simulink model "bh_compare_hand_to_SM_quad_pend"  (R2021b)
settings: Solver=ode23t  StartTime=0.0  StopTime=50  FixedStep=0.001  RelTol=1e-5  EnableMultiTasking=on
values from neighbouring files (symbols this model uses):
  K = [0.0865712753524 0.00277244570809 -0.0192153083791 -0.00162453351485 3.32348361895e-08 -1.41900444311e-08 -0.0932413563659 2.38058592401e-06 6.56188614095e-09 -0.0932413743514 2.52459639721e-09 9.53911962763e-08 ... (84 elements, 4x21)]    [CONFIRMED_bh_CONT_DES_RESULTS.mat]    (also in CONFIRMED_bh_CONT_DES_RESULTS_DISCRETE.mat = [-4.44584196463e-19 1.60298866655e-18 6.22915677006e-18 0 -9; CONFIRMED_bh_CONT_DES_RESULTS_DISCRETE_PRE_19a_using_DARE_SOLVER.mat = [-0.000193022438438 0.000285510081841 0.000531074046333 0.00; CONFIRMED_bh_CONT_DES_RESULTS_DISCRETE_R2019b.mat = [3.0073494701e-20 1.31173839205e-18 -5.80308139081e-19 0 8.7; CONFIRMED_bh_CONT_DES_RESULTS_PRE_19a_using_CARE_SOLVER.mat = [3.8473936011e-07 5.10337913269e-05 5.50269068807e-05 0.0072)
  xme_dot_0 = (bRg .') * Vm_0(:)    [bh_func_for_lagr_mask_init.m]
undefined symbols (not defined in the file or in its folder): P_elec, P_mot, P_one_prop, P_pend, P_rot, P_veh, P_veh_no_props, sigbuilder_block, X, Y, Z
libraries: fl_lib x85, simulink_extras x42, nesl_utility x39, sm_lib x29, bh_6dof_LIBRARY x22, slpidlib x8, fl_ps_legacy_lib x7, simulink x2
(part 4 of 5)

== system bh_compare_hand_to_SM_quad_pend/MODEL_SYS/bh_6DOF (Simscape)/6DOF_JOINT_SYS/Angular_MEAS ==
  note: NOTE:  For the Transform sensor  block
      | Tthe DCM is:   r_BASE = R * r_FOLLOWER
  note: NOTE:  For the Transform sensor  block
      | The angular velocities are resolved into FOLLOWER frame components
  Calc Euler_rates : Subsystem
  Gain : Gain
  Math Function : Math  Operator=transpose  SignedPower=on  SaturateOnIntegerOverflow=on
  Mux : Mux  Inputs=3
  PS-Simulink Converter1 : nesl_utility/PS-Simulink Converter  PhysicalDomain=network_engine_domain  SubClassName=ps_output  LeftPortType=input  RightPortType=output  PseudoPeriodic=off  Frequencies=[]  Unit=rad/s  AffineConversion=off
      settings: SourceProductBaseCode=PW,SS
  PS-Simulink Converter2 : nesl_utility/PS-Simulink Converter  PhysicalDomain=network_engine_domain  SubClassName=ps_output  LeftPortType=input  RightPortType=output  PseudoPeriodic=off  Frequencies=[]  Unit=rad/s  AffineConversion=off
      settings: SourceProductBaseCode=PW,SS
  PS-Simulink Converter6 : nesl_utility/PS-Simulink Converter  PhysicalDomain=network_engine_domain  SubClassName=ps_output  LeftPortType=input  RightPortType=output  PseudoPeriodic=off  Frequencies=[]  Unit=1  AffineConversion=off
      settings: SourceProductBaseCode=PW,SS
  PS-Simulink Converter7 : nesl_utility/PS-Simulink Converter  PhysicalDomain=network_engine_domain  SubClassName=ps_output  LeftPortType=input  RightPortType=output  PseudoPeriodic=off  Frequencies=[]  Unit=rad/s  AffineConversion=off
      settings: SourceProductBaseCode=PW,SS
  Reshape1 : Reshape  OutputDimensionality=Column vector (2-D)
  Reshape2 : Reshape  OutputDimensionality=Column vector (2-D)
  Reshape3 : Reshape  OutputDimensionality=Column vector (2-D)
  Transform Sensor : sm_lib/Frames and Transforms/Transform Sensor  MeasurementFrame=Base  SenseAngle=off  SenseAxis=off  SenseAngle1=off  SenseAngle2=off  SenseAngle3=off  SenseQ=off  SenseR=on  SenseOmegaX=off  SenseOmegaY=off  SenseOmegaZ=off  SenseOmega1=off  SenseOmega2=off  SenseOmega3=off  SenseQDot=off  SenseRDot=off  SenseAlphaX=off  SenseAlphaY=off  SenseAlphaZ=off  SenseAlpha1=off  SenseAlpha2=off  SenseAlpha3=off  SenseQDDot=off  SenseRDDot=off  SenseX=off  SenseY=off  SenseZ=off  SenseRad=off  SenseAzim=off  SenseDist=off  SenseInc=off  SenseXDot=off  SenseYDot=off  SenseZDot=off  SenseRadDot=off  SenseAzimDot=off  SenseDistDot=off  SenseIncDot=off  SenseXDDot=off  SenseYDDot=off  SenseZDDot=off  SenseRadDDot=off  SenseAzimDDot=off  SenseDistDDot=off  SenseIncDDot=off
  Transform Sensor1 : sm_lib/Frames and Transforms/Transform Sensor  MeasurementFrame=Follower  SenseAngle=off  SenseAxis=off  SenseAngle1=off  SenseAngle2=off  SenseAngle3=off  SenseQ=off  SenseR=off  SenseOmegaX=on  SenseOmegaY=on  SenseOmegaZ=on  SenseOmega1=off  SenseOmega2=off  SenseOmega3=off  SenseQDot=off  SenseRDot=off  SenseAlphaX=off  SenseAlphaY=off  SenseAlphaZ=off  SenseAlpha1=off  SenseAlpha2=off  SenseAlpha3=off  SenseQDDot=off  SenseRDDot=off  SenseX=off  SenseY=off  SenseZ=off  SenseRad=off  SenseAzim=off  SenseDist=off  SenseInc=off  SenseXDot=off  SenseYDot=off  SenseZDot=off  SenseRadDot=off  SenseAzimDot=off  SenseDistDot=off  SenseIncDot=off  SenseXDDot=off  SenseYDDot=off  SenseZDDot=off  SenseRadDDot=off  SenseAzimDDot=off  SenseDistDDot=off  SenseIncDDot=off
  calc_DCM : MATLAB Function  TreatAsAtomicUnit=on
  B : PMIOPort  Side=Left
  F : PMIOPort  Port=2  Side=Right
  wb : Outport  VectorParamsAs1DForOutWhenUnconnected=off
  bRg : Outport  Port=2  VectorParamsAs1DForOutWhenUnconnected=off
  eul : Outport  Port=3  VectorParamsAs1DForOutWhenUnconnected=off
  eul_rates : Outport  Port=4  VectorParamsAs1DForOutWhenUnconnected=off
  wires:
  PS-Simulink Converter6/1 -> Gain/1  "BRF"
  PS-Simulink Converter7/1 -> Mux/1
  PS-Simulink Converter1/1 -> Mux/2
  PS-Simulink Converter2/1 -> Mux/3
  Gain/1 -> Math Function/1  "gRb"
  Math Function/1 -> [bRg], bRg/1  "bRg"
  Mux/1 -> Reshape1/1
  [bRg] -> calc_DCM/1(bRg)
  calc_DCM/1(eul_vec) -> Reshape2/1
  Reshape2/1 -> [e], eul/1
  Calc Euler_rates/1(Euler_rates) -> Reshape3/1
  Reshape3/1 -> eul_rates/1
  Reshape1/1 -> [wb], wb/1
  [wb] -> Calc Euler_rates/1("p q r ")
  [e] -> Calc Euler_rates/2(Euler_angs)
  connections:
  PS-Simulink Converter7/LConn1 -- Transform Sensor1/RConn2
  PS-Simulink Converter6/LConn1 -- Transform Sensor/RConn2
  Transform Sensor1/RConn1 -- Transform Sensor/RConn1 -- F/RConn1
  Transform Sensor/LConn1 -- B/RConn1 -- Transform Sensor1/LConn1
  PS-Simulink Converter2/LConn1 -- Transform Sensor1/RConn4
  Transform Sensor1/RConn3 -- PS-Simulink Converter1/LConn1

== system bh_compare_hand_to_SM_quad_pend/MODEL_SYS/bh_6DOF (Simscape)/PEND_SYS/Pend_Angular_MEAS ==
  note: NOTE:  For the Transform sensor  block
      | Tthe DCM is:   r_BASE = R * r_FOLLOWER
  note: NOTE:  For the Transform sensor  block
      | The angular velocities are resolved into FOLLOWER frame components
  Calc Euler_rates : Subsystem
  Gain : Gain
  Math Function : Math  Operator=transpose  SignedPower=on  SaturateOnIntegerOverflow=on
  Mux : Mux  Inputs=3
  PS-Simulink Converter1 : nesl_utility/PS-Simulink Converter  PhysicalDomain=network_engine_domain  SubClassName=ps_output  LeftPortType=input  RightPortType=output  PseudoPeriodic=off  Frequencies=[]  Unit=rad/s  AffineConversion=off
      settings: SourceProductBaseCode=PW,SS
  PS-Simulink Converter2 : nesl_utility/PS-Simulink Converter  PhysicalDomain=network_engine_domain  SubClassName=ps_output  LeftPortType=input  RightPortType=output  PseudoPeriodic=off  Frequencies=[]  Unit=rad/s  AffineConversion=off
      settings: SourceProductBaseCode=PW,SS
  PS-Simulink Converter6 : nesl_utility/PS-Simulink Converter  PhysicalDomain=network_engine_domain  SubClassName=ps_output  LeftPortType=input  RightPortType=output  PseudoPeriodic=off  Frequencies=[]  Unit=1  AffineConversion=off
      settings: SourceProductBaseCode=PW,SS
  PS-Simulink Converter7 : nesl_utility/PS-Simulink Converter  PhysicalDomain=network_engine_domain  SubClassName=ps_output  LeftPortType=input  RightPortType=output  PseudoPeriodic=off  Frequencies=[]  Unit=rad/s  AffineConversion=off
      settings: SourceProductBaseCode=PW,SS
  Reshape1 : Reshape  OutputDimensionality=Column vector (2-D)
  Reshape2 : Reshape  OutputDimensionality=Column vector (2-D)
  Reshape3 : Reshape  OutputDimensionality=Column vector (2-D)
  Transform Sensor : sm_lib/Frames and Transforms/Transform Sensor  MeasurementFrame=Base  SenseAngle=off  SenseAxis=off  SenseAngle1=off  SenseAngle2=off  SenseAngle3=off  SenseQ=off  SenseR=on  SenseOmegaX=off  SenseOmegaY=off  SenseOmegaZ=off  SenseOmega1=off  SenseOmega2=off  SenseOmega3=off  SenseQDot=off  SenseRDot=off  SenseAlphaX=off  SenseAlphaY=off  SenseAlphaZ=off  SenseAlpha1=off  SenseAlpha2=off  SenseAlpha3=off  SenseQDDot=off  SenseRDDot=off  SenseX=off  SenseY=off  SenseZ=off  SenseRad=off  SenseAzim=off  SenseDist=off  SenseInc=off  SenseXDot=off  SenseYDot=off  SenseZDot=off  SenseRadDot=off  SenseAzimDot=off  SenseDistDot=off  SenseIncDot=off  SenseXDDot=off  SenseYDDot=off  SenseZDDot=off  SenseRadDDot=off  SenseAzimDDot=off  SenseDistDDot=off  SenseIncDDot=off
  Transform Sensor1 : sm_lib/Frames and Transforms/Transform Sensor  MeasurementFrame=Follower  SenseAngle=off  SenseAxis=off  SenseAngle1=off  SenseAngle2=off  SenseAngle3=off  SenseQ=off  SenseR=off  SenseOmegaX=on  SenseOmegaY=on  SenseOmegaZ=on  SenseOmega1=off  SenseOmega2=off  SenseOmega3=off  SenseQDot=off  SenseRDot=off  SenseAlphaX=off  SenseAlphaY=off  SenseAlphaZ=off  SenseAlpha1=off  SenseAlpha2=off  SenseAlpha3=off  SenseQDDot=off  SenseRDDot=off  SenseX=off  SenseY=off  SenseZ=off  SenseRad=off  SenseAzim=off  SenseDist=off  SenseInc=off  SenseXDot=off  SenseYDot=off  SenseZDot=off  SenseRadDot=off  SenseAzimDot=off  SenseDistDot=off  SenseIncDot=off  SenseXDDot=off  SenseYDDot=off  SenseZDDot=off  SenseRadDDot=off  SenseAzimDDot=off  SenseDistDDot=off  SenseIncDDot=off
      settings: AttributesFormatString=MeasComponentFrame = %<MeasurementFrame>
  calc_DCM : MATLAB Function  TreatAsAtomicUnit=on
  V : PMIOPort  Side=Left
  P : PMIOPort  Port=2  Side=Right
  wb : Outport  VectorParamsAs1DForOutWhenUnconnected=off
  bRg : Outport  Port=2  VectorParamsAs1DForOutWhenUnconnected=off
  eul : Outport  Port=3  VectorParamsAs1DForOutWhenUnconnected=off
  eul_rates : Outport  Port=4  VectorParamsAs1DForOutWhenUnconnected=off
  wires:
  PS-Simulink Converter6/1 -> Gain/1  "BRF"
  PS-Simulink Converter7/1 -> Mux/1
  PS-Simulink Converter1/1 -> Mux/2
  PS-Simulink Converter2/1 -> Mux/3
  Gain/1 -> Math Function/1  "gRb"
  Math Function/1 -> [bRg], bRg/1  "bRg"
  Mux/1 -> Reshape1/1
  [bRg] -> calc_DCM/1(bRg)
  calc_DCM/1(eul_vec) -> Reshape2/1
  Reshape2/1 -> [e], eul/1
  Calc Euler_rates/1(Euler_rates) -> Reshape3/1
  Reshape3/1 -> eul_rates/1
  Reshape1/1 -> [wb], wb/1
  [wb] -> Calc Euler_rates/1("p q r ")
  [e] -> Calc Euler_rates/2(Euler_angs)
  connections:
  PS-Simulink Converter7/LConn1 -- Transform Sensor1/RConn2
  PS-Simulink Converter6/LConn1 -- Transform Sensor/RConn2
  Transform Sensor1/RConn1 -- Transform Sensor/RConn1 -- P/RConn1
  Transform Sensor/LConn1 -- V/RConn1 -- Transform Sensor1/LConn1
  PS-Simulink Converter2/LConn1 -- Transform Sensor1/RConn4
  Transform Sensor1/RConn3 -- PS-Simulink Converter1/LConn1

== system bh_compare_hand_to_SM_quad_pend/MODEL_SYS/bh_6DOF (Simscape)/Propellers/MOT_AERO_PROP_1 ==
  w_CMD_signed : Inport
  Abs : Abs  Commented=on
  Abs1 : Abs  Commented=on
  Bus Creator : BusCreator  Inputs=3
  DRAQ_and_Thrust_on_PROP : Subsystem
  External Force and Torque : sm_lib/Forces and Torques/External Force and Torque  ForceResolutionFrame=AttachedFrame  EnableForceX=off  EnableForceY=off  EnableForceZ=on  EnableForce=off  TorqueResolutionFrame=AttachedFrame  EnableTorqueX=off  EnableTorqueY=off  EnableTorqueZ=on  EnableTorque=off
  From : From  Commented=on  GotoTag=TQ_prop
  From4 : From  Commented=on  GotoTag=TQ_veh
  From5 : From  Commented=on  GotoTag=w_prop
  Gain1 : Gain  Commented=on  Gain=P_mot.b
  Mux : Mux  Commented=on  Inputs=2
  PS-Simulink Converter1 : nesl_utility/PS-Simulink Converter  PhysicalDomain=network_engine_domain  SubClassName=ps_output  LeftPortType=input  RightPortType=output  PseudoPeriodic=off  Frequencies=[]  Unit=rad/s  AffineConversion=off
      settings: SourceProductBaseCode=PW,SS
  PS-Simulink Converter2 : nesl_utility/PS-Simulink Converter  PhysicalDomain=network_engine_domain  SubClassName=ps_output  LeftPortType=input  RightPortType=output  PseudoPeriodic=off  Frequencies=[]  Unit=N*m  AffineConversion=off
      settings: SourceProductBaseCode=PW,SS
  Scope : Scope  Commented=on  NumInputPorts=2
  Selector : Selector  InputPortWidth=3  IndexOptions=Index vector (dialog)  Indices=3  OutputSizes=1
  TQ_on_propeller : Subsystem
  joint_prop : sm_lib/Joints/Revolute Joint  JointMode=Normal  SenseConstraintForce=off  SenseConstraintForceX=off  SenseConstraintForceY=off  SenseConstraintForceZ=off  SenseConstraintTorque=off  SenseConstraintTorqueX=off  SenseConstraintTorqueY=off  SenseConstraintTorqueZ=off  SenseTotalForce=off  SenseTotalForceX=off  SenseTotalForceY=off  SenseTotalForceZ=off  SenseTotalTorque=on  SenseTotalTorqueX=off  SenseTotalTorqueY=off  SenseTotalTorqueZ=off  CompositeWrenchDir=FollowerOnBase  CompositeWrenchFrame=BaseFrame  EquilibriumPosition=0  EquilibriumPositionUnits=deg  SpringStiffness=0  SpringStiffnessUnits=N*m/deg  DampingCoefficient=P_mot.b  DampingCoefficientUnits=N*m/(rad/s)  TorqueActuationMode=InputTorque  MotionActuationMode=ComputedMotion  SensePosition=off  SenseVelocity=on  SenseAcceleration=off  SenseTorqueForce=off  SenseLowerLimitTorqueForce=off  SenseUpperLimitTorqueForce=off  LowerLimitSpecify=off  LowerLimitBound=-90  LowerLimitBoundUnits=deg  LowerLimitStiffness=1e4  LowerLimitStiffnessUnits=N*m/deg  LowerLimitDamping=10  LowerLimitDampingUnits=N*m/(deg/s)  LowerLimitTransitionRegionWidth=0.1  LowerLimitTransitionRegionWidthUnits=deg  UpperLimitSpecify=off  UpperLimitBound=90  UpperLimitBoundUnits=deg  UpperLimitStiffness=1e4  UpperLimitStiffnessUnits=N*m/deg  UpperLimitDamping=10  UpperLimitDampingUnits=N*m/(deg/s)  UpperLimitTransitionRegionWidth=0.1  UpperLimitTransitionRegionWidthUnits=deg  PositionTargetSpecify=off  PositionTargetPriority=High  PositionTargetValue=0  PositionTargetValueUnits=deg  VelocityTargetSpecify=off  VelocityTargetPriority=High  VelocityTargetValue=0  VelocityTargetValueUnits=deg/s
      settings: AttributesFormatString=DAMP = %<DampingCoefficient> %<DampingCoefficientUnits>
  "AirFrame " : PMIOPort  Side=Left
  PROP : PMIOPort  Port=2  Side=Right
  prop_BUS : Outport  VectorParamsAs1DForOutWhenUnconnected=off
  wires:
  w_CMD_signed/1 -> TQ_on_propeller/1(w_CMD_signed)
  TQ_on_propeller/1(TQ_Ki) -> [TQ_prop]
  DRAQ_and_Thrust_on_PROP/1(TH_veh) -> [TH_veh]
  PS-Simulink Converter1/1 -> [w_prop]
  [TH_veh] -> Bus Creator/1  "Thrust_on_veh"
  [w_prop] -> Bus Creator/3  "w_prop"
  [TQ_veh] -> Bus Creator/2  "Torque_on_veh"
  Bus Creator/1 -> prop_BUS/1
  Selector/1 -> [TQ_veh]
  PS-Simulink Converter2/1 -> Selector/1
  Mux/1 -> Scope/1
  From/1 -> Abs1/1
  From4/1 -> Abs/1
  Abs/1 -> Mux/1
  Abs1/1 -> Mux/2
  Gain1/1 -> Scope/2
  From5/1 -> Gain1/1
  connections:
  joint_prop/RConn2 -- DRAQ_and_Thrust_on_PROP/LConn1 -- TQ_on_propeller/LConn1 -- PS-Simulink Converter1/LConn1
  TQ_on_propeller/RConn1 -- joint_prop/LConn2
  External Force and Torque/RConn1 -- joint_prop/RConn1 -- PROP/RConn1
  DRAQ_and_Thrust_on_PROP/RConn2 -- External Force and Torque/LConn2
  DRAQ_and_Thrust_on_PROP/RConn1 -- External Force and Torque/LConn1
  "AirFrame "/RConn1 -- joint_prop/LConn1
  PS-Simulink Converter2/LConn1 -- joint_prop/RConn3

== system bh_compare_hand_to_SM_quad_pend/MODEL_SYS/bh_6DOF (Simscape)/Propellers/MOT_AERO_PROP_2 ==
  w_CMD_signed : Inport
  Abs : Abs  Commented=on
  Abs1 : Abs  Commented=on
  Bus Creator : BusCreator  Inputs=3
  DRAQ_and_Thrust_on_PROP : Subsystem
  External Force and Torque : sm_lib/Forces and Torques/External Force and Torque  ForceResolutionFrame=AttachedFrame  EnableForceX=off  EnableForceY=off  EnableForceZ=on  EnableForce=off  TorqueResolutionFrame=AttachedFrame  EnableTorqueX=off  EnableTorqueY=off  EnableTorqueZ=on  EnableTorque=off
  From : From  Commented=on  GotoTag=TQ_prop
  From4 : From  Commented=on  GotoTag=TQ_veh
  From5 : From  Commented=on  GotoTag=w_prop
  Gain1 : Gain  Commented=on  Gain=P_mot.b
  Mux : Mux  Commented=on  Inputs=2
  PS-Simulink Converter1 : nesl_utility/PS-Simulink Converter  PhysicalDomain=network_engine_domain  SubClassName=ps_output  LeftPortType=input  RightPortType=output  PseudoPeriodic=off  Frequencies=[]  Unit=rad/s  AffineConversion=off
      settings: SourceProductBaseCode=PW,SS
  PS-Simulink Converter2 : nesl_utility/PS-Simulink Converter  PhysicalDomain=network_engine_domain  SubClassName=ps_output  LeftPortType=input  RightPortType=output  PseudoPeriodic=off  Frequencies=[]  Unit=N*m  AffineConversion=off
      settings: SourceProductBaseCode=PW,SS
  Scope : Scope  Commented=on  NumInputPorts=2
  Selector : Selector  InputPortWidth=3  IndexOptions=Index vector (dialog)  Indices=3  OutputSizes=1
  TQ_on_propeller : Subsystem
  joint_prop : sm_lib/Joints/Revolute Joint  JointMode=Normal  SenseConstraintForce=off  SenseConstraintForceX=off  SenseConstraintForceY=off  SenseConstraintForceZ=off  SenseConstraintTorque=off  SenseConstraintTorqueX=off  SenseConstraintTorqueY=off  SenseConstraintTorqueZ=off  SenseTotalForce=off  SenseTotalForceX=off  SenseTotalForceY=off  SenseTotalForceZ=off  SenseTotalTorque=on  SenseTotalTorqueX=off  SenseTotalTorqueY=off  SenseTotalTorqueZ=off  CompositeWrenchDir=FollowerOnBase  CompositeWrenchFrame=BaseFrame  EquilibriumPosition=0  EquilibriumPositionUnits=deg  SpringStiffness=0  SpringStiffnessUnits=N*m/deg  DampingCoefficient=P_mot.b  DampingCoefficientUnits=N*m/(rad/s)  TorqueActuationMode=InputTorque  MotionActuationMode=ComputedMotion  SensePosition=off  SenseVelocity=on  SenseAcceleration=off  SenseTorqueForce=off  SenseLowerLimitTorqueForce=off  SenseUpperLimitTorqueForce=off  LowerLimitSpecify=off  LowerLimitBound=-90  LowerLimitBoundUnits=deg  LowerLimitStiffness=1e4  LowerLimitStiffnessUnits=N*m/deg  LowerLimitDamping=10  LowerLimitDampingUnits=N*m/(deg/s)  LowerLimitTransitionRegionWidth=0.1  LowerLimitTransitionRegionWidthUnits=deg  UpperLimitSpecify=off  UpperLimitBound=90  UpperLimitBoundUnits=deg  UpperLimitStiffness=1e4  UpperLimitStiffnessUnits=N*m/deg  UpperLimitDamping=10  UpperLimitDampingUnits=N*m/(deg/s)  UpperLimitTransitionRegionWidth=0.1  UpperLimitTransitionRegionWidthUnits=deg  PositionTargetSpecify=off  PositionTargetPriority=High  PositionTargetValue=0  PositionTargetValueUnits=deg  VelocityTargetSpecify=off  VelocityTargetPriority=High  VelocityTargetValue=0  VelocityTargetValueUnits=deg/s
      settings: AttributesFormatString=DAMP = %<DampingCoefficient> %<DampingCoefficientUnits>
  "AirFrame " : PMIOPort  Side=Left
  PROP : PMIOPort  Port=2  Side=Right
  prop_BUS : Outport  VectorParamsAs1DForOutWhenUnconnected=off
  wires:
  w_CMD_signed/1 -> TQ_on_propeller/1(w_CMD_signed)
  TQ_on_propeller/1(TQ_Ki) -> [TQ_prop]
  DRAQ_and_Thrust_on_PROP/1(TH_veh) -> [TH_veh]
  PS-Simulink Converter1/1 -> [w_prop]
  [TH_veh] -> Bus Creator/1  "Thrust_on_veh"
  [w_prop] -> Bus Creator/3  "w_prop"
  [TQ_veh] -> Bus Creator/2  "Torque_on_veh"
  Bus Creator/1 -> prop_BUS/1
  Selector/1 -> [TQ_veh]
  PS-Simulink Converter2/1 -> Selector/1
  Mux/1 -> Scope/1
  From/1 -> Abs1/1
  From4/1 -> Abs/1
  Abs/1 -> Mux/1
  Abs1/1 -> Mux/2
  Gain1/1 -> Scope/2
  From5/1 -> Gain1/1
  connections:
  TQ_on_propeller/LConn1 -- PS-Simulink Converter1/LConn1 -- DRAQ_and_Thrust_on_PROP/LConn1 -- joint_prop/RConn2
  TQ_on_propeller/RConn1 -- joint_prop/LConn2
  External Force and Torque/RConn1 -- joint_prop/RConn1 -- PROP/RConn1
  DRAQ_and_Thrust_on_PROP/RConn2 -- External Force and Torque/LConn2
  DRAQ_and_Thrust_on_PROP/RConn1 -- External Force and Torque/LConn1
  "AirFrame "/RConn1 -- joint_prop/LConn1
  PS-Simulink Converter2/LConn1 -- joint_prop/RConn3

== system bh_compare_hand_to_SM_quad_pend/MODEL_SYS/bh_6DOF (Simscape)/Propellers/MOT_AERO_PROP_3 ==
  w_CMD_signed : Inport
  Abs : Abs  Commented=on
  Abs1 : Abs  Commented=on
  Bus Creator : BusCreator  Inputs=3
  DRAQ_and_Thrust_on_PROP : Subsystem
  External Force and Torque : sm_lib/Forces and Torques/External Force and Torque  ForceResolutionFrame=AttachedFrame  EnableForceX=off  EnableForceY=off  EnableForceZ=on  EnableForce=off  TorqueResolutionFrame=AttachedFrame  EnableTorqueX=off  EnableTorqueY=off  EnableTorqueZ=on  EnableTorque=off
  From : From  Commented=on  GotoTag=TQ_prop
  From4 : From  Commented=on  GotoTag=TQ_veh
  From5 : From  Commented=on  GotoTag=w_prop
  Gain1 : Gain  Commented=on  Gain=P_mot.b
  Mux : Mux  Commented=on  Inputs=2
  PS-Simulink Converter1 : nesl_utility/PS-Simulink Converter  PhysicalDomain=network_engine_domain  SubClassName=ps_output  LeftPortType=input  RightPortType=output  PseudoPeriodic=off  Frequencies=[]  Unit=rad/s  AffineConversion=off
      settings: SourceProductBaseCode=PW,SS
  PS-Simulink Converter2 : nesl_utility/PS-Simulink Converter  PhysicalDomain=network_engine_domain  SubClassName=ps_output  LeftPortType=input  RightPortType=output  PseudoPeriodic=off  Frequencies=[]  Unit=N*m  AffineConversion=off
      settings: SourceProductBaseCode=PW,SS
  Scope : Scope  Commented=on  NumInputPorts=2
  Selector : Selector  InputPortWidth=3  IndexOptions=Index vector (dialog)  Indices=3  OutputSizes=1
  TQ_on_propeller : Subsystem
  joint_prop : sm_lib/Joints/Revolute Joint  JointMode=Normal  SenseConstraintForce=off  SenseConstraintForceX=off  SenseConstraintForceY=off  SenseConstraintForceZ=off  SenseConstraintTorque=off  SenseConstraintTorqueX=off  SenseConstraintTorqueY=off  SenseConstraintTorqueZ=off  SenseTotalForce=off  SenseTotalForceX=off  SenseTotalForceY=off  SenseTotalForceZ=off  SenseTotalTorque=on  SenseTotalTorqueX=off  SenseTotalTorqueY=off  SenseTotalTorqueZ=off  CompositeWrenchDir=FollowerOnBase  CompositeWrenchFrame=BaseFrame  EquilibriumPosition=0  EquilibriumPositionUnits=deg  SpringStiffness=0  SpringStiffnessUnits=N*m/deg  DampingCoefficient=P_mot.b  DampingCoefficientUnits=N*m/(rad/s)  TorqueActuationMode=InputTorque  MotionActuationMode=ComputedMotion  SensePosition=off  SenseVelocity=on  SenseAcceleration=off  SenseTorqueForce=off  SenseLowerLimitTorqueForce=off  SenseUpperLimitTorqueForce=off  LowerLimitSpecify=off  LowerLimitBound=-90  LowerLimitBoundUnits=deg  LowerLimitStiffness=1e4  LowerLimitStiffnessUnits=N*m/deg  LowerLimitDamping=10  LowerLimitDampingUnits=N*m/(deg/s)  LowerLimitTransitionRegionWidth=0.1  LowerLimitTransitionRegionWidthUnits=deg  UpperLimitSpecify=off  UpperLimitBound=90  UpperLimitBoundUnits=deg  UpperLimitStiffness=1e4  UpperLimitStiffnessUnits=N*m/deg  UpperLimitDamping=10  UpperLimitDampingUnits=N*m/(deg/s)  UpperLimitTransitionRegionWidth=0.1  UpperLimitTransitionRegionWidthUnits=deg  PositionTargetSpecify=off  PositionTargetPriority=High  PositionTargetValue=0  PositionTargetValueUnits=deg  VelocityTargetSpecify=off  VelocityTargetPriority=High  VelocityTargetValue=0  VelocityTargetValueUnits=deg/s
      settings: AttributesFormatString=DAMP = %<DampingCoefficient> %<DampingCoefficientUnits>
  "AirFrame " : PMIOPort  Side=Left
  PROP : PMIOPort  Port=2  Side=Right
  prop_BUS : Outport  VectorParamsAs1DForOutWhenUnconnected=off
  wires:
  w_CMD_signed/1 -> TQ_on_propeller/1(w_CMD_signed)
  TQ_on_propeller/1(TQ_Ki) -> [TQ_prop]
  DRAQ_and_Thrust_on_PROP/1(TH_veh) -> [TH_veh]
  PS-Simulink Converter1/1 -> [w_prop]
  [TH_veh] -> Bus Creator/1  "Thrust_on_veh"
  [w_prop] -> Bus Creator/3  "w_prop"
  [TQ_veh] -> Bus Creator/2  "Torque_on_veh"
  Bus Creator/1 -> prop_BUS/1
  Selector/1 -> [TQ_veh]
  PS-Simulink Converter2/1 -> Selector/1
  Mux/1 -> Scope/1
  From/1 -> Abs1/1
  From4/1 -> Abs/1
  Abs/1 -> Mux/1
  Abs1/1 -> Mux/2
  Gain1/1 -> Scope/2
  From5/1 -> Gain1/1
  connections:
  TQ_on_propeller/LConn1 -- PS-Simulink Converter1/LConn1 -- DRAQ_and_Thrust_on_PROP/LConn1 -- joint_prop/RConn2
  TQ_on_propeller/RConn1 -- joint_prop/LConn2
  External Force and Torque/RConn1 -- joint_prop/RConn1 -- PROP/RConn1
  DRAQ_and_Thrust_on_PROP/RConn2 -- External Force and Torque/LConn2
  DRAQ_and_Thrust_on_PROP/RConn1 -- External Force and Torque/LConn1
  "AirFrame "/RConn1 -- joint_prop/LConn1
  PS-Simulink Converter2/LConn1 -- joint_prop/RConn3

== system bh_compare_hand_to_SM_quad_pend/MODEL_SYS/bh_6DOF (Simscape)/Propellers/MOT_AERO_PROP_4 ==
  w_CMD_signed : Inport
  Abs : Abs  Commented=on
  Abs1 : Abs  Commented=on
  Bus Creator : BusCreator  Inputs=3
  DRAQ_and_Thrust_on_PROP : Subsystem
  External Force and Torque : sm_lib/Forces and Torques/External Force and Torque  ForceResolutionFrame=AttachedFrame  EnableForceX=off  EnableForceY=off  EnableForceZ=on  EnableForce=off  TorqueResolutionFrame=AttachedFrame  EnableTorqueX=off  EnableTorqueY=off  EnableTorqueZ=on  EnableTorque=off
  From : From  Commented=on  GotoTag=TQ_prop
  From4 : From  Commented=on  GotoTag=TQ_veh
  From5 : From  Commented=on  GotoTag=w_prop
  Gain1 : Gain  Commented=on  Gain=P_mot.b
  Mux : Mux  Commented=on  Inputs=2
  PS-Simulink Converter1 : nesl_utility/PS-Simulink Converter  PhysicalDomain=network_engine_domain  SubClassName=ps_output  LeftPortType=input  RightPortType=output  PseudoPeriodic=off  Frequencies=[]  Unit=rad/s  AffineConversion=off
      settings: SourceProductBaseCode=PW,SS
  PS-Simulink Converter2 : nesl_utility/PS-Simulink Converter  PhysicalDomain=network_engine_domain  SubClassName=ps_output  LeftPortType=input  RightPortType=output  PseudoPeriodic=off  Frequencies=[]  Unit=N*m  AffineConversion=off
      settings: SourceProductBaseCode=PW,SS
  Scope : Scope  Commented=on  NumInputPorts=2
  Selector : Selector  InputPortWidth=3  IndexOptions=Index vector (dialog)  Indices=3  OutputSizes=1
  TQ_on_propeller : Subsystem
  joint_prop : sm_lib/Joints/Revolute Joint  JointMode=Normal  SenseConstraintForce=off  SenseConstraintForceX=off  SenseConstraintForceY=off  SenseConstraintForceZ=off  SenseConstraintTorque=off  SenseConstraintTorqueX=off  SenseConstraintTorqueY=off  SenseConstraintTorqueZ=off  SenseTotalForce=off  SenseTotalForceX=off  SenseTotalForceY=off  SenseTotalForceZ=off  SenseTotalTorque=on  SenseTotalTorqueX=off  SenseTotalTorqueY=off  SenseTotalTorqueZ=off  CompositeWrenchDir=FollowerOnBase  CompositeWrenchFrame=BaseFrame  EquilibriumPosition=0  EquilibriumPositionUnits=deg  SpringStiffness=0  SpringStiffnessUnits=N*m/deg  DampingCoefficient=P_mot.b  DampingCoefficientUnits=N*m/(rad/s)  TorqueActuationMode=InputTorque  MotionActuationMode=ComputedMotion  SensePosition=off  SenseVelocity=on  SenseAcceleration=off  SenseTorqueForce=off  SenseLowerLimitTorqueForce=off  SenseUpperLimitTorqueForce=off  LowerLimitSpecify=off  LowerLimitBound=-90  LowerLimitBoundUnits=deg  LowerLimitStiffness=1e4  LowerLimitStiffnessUnits=N*m/deg  LowerLimitDamping=10  LowerLimitDampingUnits=N*m/(deg/s)  LowerLimitTransitionRegionWidth=0.1  LowerLimitTransitionRegionWidthUnits=deg  UpperLimitSpecify=off  UpperLimitBound=90  UpperLimitBoundUnits=deg  UpperLimitStiffness=1e4  UpperLimitStiffnessUnits=N*m/deg  UpperLimitDamping=10  UpperLimitDampingUnits=N*m/(deg/s)  UpperLimitTransitionRegionWidth=0.1  UpperLimitTransitionRegionWidthUnits=deg  PositionTargetSpecify=off  PositionTargetPriority=High  PositionTargetValue=0  PositionTargetValueUnits=deg  VelocityTargetSpecify=off  VelocityTargetPriority=High  VelocityTargetValue=0  VelocityTargetValueUnits=deg/s
      settings: AttributesFormatString=DAMP = %<DampingCoefficient> %<DampingCoefficientUnits>
  "AirFrame " : PMIOPort  Side=Left
  PROP : PMIOPort  Port=2  Side=Right
  prop_BUS : Outport  VectorParamsAs1DForOutWhenUnconnected=off
  wires:
  w_CMD_signed/1 -> TQ_on_propeller/1(w_CMD_signed)
  TQ_on_propeller/1(TQ_Ki) -> [TQ_prop]
  DRAQ_and_Thrust_on_PROP/1(TH_veh) -> [TH_veh]
  PS-Simulink Converter1/1 -> [w_prop]
  [TH_veh] -> Bus Creator/1  "Thrust_on_veh"
  [w_prop] -> Bus Creator/3  "w_prop"
  [TQ_veh] -> Bus Creator/2  "Torque_on_veh"
  Bus Creator/1 -> prop_BUS/1
  Selector/1 -> [TQ_veh]
  PS-Simulink Converter2/1 -> Selector/1
  Mux/1 -> Scope/1
  From/1 -> Abs1/1
  From4/1 -> Abs/1
  Abs/1 -> Mux/1
  Abs1/1 -> Mux/2
  Gain1/1 -> Scope/2
  From5/1 -> Gain1/1
  connections:
  TQ_on_propeller/LConn1 -- PS-Simulink Converter1/LConn1 -- joint_prop/RConn2 -- DRAQ_and_Thrust_on_PROP/LConn1
  TQ_on_propeller/RConn1 -- joint_prop/LConn2
  External Force and Torque/RConn1 -- joint_prop/RConn1 -- PROP/RConn1
  External Force and Torque/LConn2 -- DRAQ_and_Thrust_on_PROP/RConn2
  External Force and Torque/LConn1 -- DRAQ_and_Thrust_on_PROP/RConn1
  "AirFrame "/RConn1 -- joint_prop/LConn1
  PS-Simulink Converter2/LConn1 -- joint_prop/RConn3

== system bh_compare_hand_to_SM_quad_pend/MODEL_SYS/bh_6DOF (Simscape)/6DOF_JOINT_SYS/Angular_MEAS/Calc Euler_rates ==
  "p q r " : Inport
  Euler_angs : Inport  Port=2
  Demux1 : Demux  Outputs=3
  Demux2 : Demux  Outputs=3
  Demux3 : Demux  Outputs=3
  Mux1 : Mux  Inputs=3
  Reshape1 : Reshape  OutputDimensionality=Column vector (2-D)
  Reshape2 : Reshape  OutputDimensionality=Column vector (2-D)
  Terminator : Terminator
  my_euler_rates : MATLAB Function  TreatAsAtomicUnit=on
  Euler_rates : Outport  VectorParamsAs1DForOutWhenUnconnected=off
  wires:
  Reshape1/1 -> Demux3/1  "wb"
  my_euler_rates/1(euler_rates) -> Demux2/1  "euler_rates"
  Demux2/3 -> Mux1/3  "psidot_X3_roll"
  Demux2/2 -> Mux1/2  "thetadot_Y2_pitch"
  Demux2/1 -> Mux1/1  "phidot_Z1_yaw"
  Reshape2/1 -> Euler_rates/1
  Mux1/1 -> Reshape2/1
  Demux3/3 -> my_euler_rates/5(r)
  Demux3/2 -> my_euler_rates/4(q)
  Demux3/1 -> my_euler_rates/3(p)
  Euler_angs/1 -> Demux1/1
  "p q r "/1 -> Reshape1/1
  Demux1/2 -> my_euler_rates/1(theta)  "theta"
  Demux1/1 -> Terminator/1  "phi"
  Demux1/3 -> my_euler_rates/2(psi)  "psi"

== system bh_compare_hand_to_SM_quad_pend/MODEL_SYS/bh_6DOF (Simscape)/PEND_SYS/Pend_Angular_MEAS/Calc Euler_rates ==
  "p q r " : Inport
  Euler_angs : Inport  Port=2
  Demux1 : Demux  Outputs=3
  Demux2 : Demux  Outputs=3
  Demux3 : Demux  Outputs=3
  Mux1 : Mux  Inputs=3
  Reshape1 : Reshape  OutputDimensionality=Column vector (2-D)
  Reshape2 : Reshape  OutputDimensionality=Column vector (2-D)
  Terminator : Terminator
  my_euler_rates : MATLAB Function  TreatAsAtomicUnit=on
  Euler_rates : Outport  VectorParamsAs1DForOutWhenUnconnected=off
  wires:
  Reshape1/1 -> Demux3/1  "wb"
  my_euler_rates/1(euler_rates) -> Demux2/1  "euler_rates"
  Demux2/3 -> Mux1/3  "psidot_X3_roll"
  Demux2/2 -> Mux1/2  "thetadot_Y2_pitch"
  Demux2/1 -> Mux1/1  "phidot_Z1_yaw"
  Reshape2/1 -> Euler_rates/1
  Mux1/1 -> Reshape2/1
  Demux3/3 -> my_euler_rates/5(r)
  Demux3/2 -> my_euler_rates/4(q)
  Demux3/1 -> my_euler_rates/3(p)
  Euler_angs/1 -> Demux1/1
  "p q r "/1 -> Reshape1/1
  Demux1/2 -> my_euler_rates/1(theta)  "theta"
  Demux1/1 -> Terminator/1  "phi"
  Demux1/3 -> my_euler_rates/2(psi)  "psi"

== system bh_compare_hand_to_SM_quad_pend/MODEL_SYS/bh_6DOF (Simscape)/Propellers/MOT_AERO_PROP_1/DRAQ_and_Thrust_on_PROP ==
  note: The "-1" is because DRAG is in the opposite direction
      | to the propeller SPIN direction
  PS Gain : fl_lib/Physical Signals/Functions/PS Gain  gain=-1
      settings: AttributesFormatString=GAIN= %<gain>
  PS Gain1 : fl_lib/Physical Signals/Functions/PS Gain  gain=P_one_prop.TWIST_per_w2 N*m/((rad/s)^2)
      settings: AttributesFormatString=GAIN= %<gain>
  PS Gain3 : fl_lib/Physical Signals/Functions/PS Gain  gain=P_one_prop.LIFT_per_w2 N/((rad/s)^2)
      settings: AttributesFormatString=GAIN= %<gain>
  PS Product : fl_lib/Physical Signals/Functions/PS Product
  PS Product1 : fl_lib/Physical Signals/Functions/PS Product
  PS Product2 : fl_lib/Physical Signals/Functions/PS Product
  PS Sign : fl_lib/Physical Signals/Nonlinear Operators/PS Sign
      settings: SourceProductBaseCode=SS  InternalSimscapePortConfiguration="{\"Bottom\":[],\"Left\":[{\"id\":\"I\",\"label\":\"\",\"type\":\"input\"}],\"Right\":[{\"id\":\"O\",\"label\":\"\",\"type\":\"output\"}],\"Top\":[]}"
  PS-Simulink Converter1 : nesl_utility/PS-Simulink Converter  PhysicalDomain=network_engine_domain  SubClassName=ps_output  LeftPortType=input  RightPortType=output  PseudoPeriodic=off  Frequencies=[]  Unit=N  AffineConversion=off
      settings: SourceProductBaseCode=PW,SS
  W : PMIOPort  Side=Left
  THRUST : PMIOPort  Port=2  Side=Right
  DRAQ_TQ : PMIOPort  Port=3  Side=Right
  TH_veh : Outport  VectorParamsAs1DForOutWhenUnconnected=off
  wires:
  PS-Simulink Converter1/1 -> TH_veh/1
  connections:
  PS Gain/LConn1 -- PS Sign/RConn1
  W/RConn1 -- PS Product/LConn1 -- PS Product/LConn2 -- PS Product2/LConn1 -- PS Product2/LConn2 -- PS Sign/LConn1
  PS Product/RConn1 -- PS Gain1/LConn1
  PS Gain1/RConn1 -- PS Product1/LConn2
  PS Gain/RConn1 -- PS Product1/LConn1
  DRAQ_TQ/RConn1 -- PS Product1/RConn1
  PS Product2/RConn1 -- PS Gain3/LConn1
  THRUST/RConn1 -- PS Gain3/RConn1 -- PS-Simulink Converter1/LConn1

== system bh_compare_hand_to_SM_quad_pend/MODEL_SYS/bh_6DOF (Simscape)/Propellers/MOT_AERO_PROP_1/TQ_on_propeller ==
  note: ATTENTION:
      | This subsystem computes the Torque that is applied to the
      | PROPELLER ... and NOT the torque applied to the airframe
  w_CMD_signed : Inport
  DC_mot_elec : Subsystem  mask(DC motor){K=P_mot.Ka, R=P_mot.R, L=P_mot.L, Kb=P_mot.Ke, ID=P_mot.ID}
      mask prompts: K "Torque constant (N.m/A)"; R "Armature resistance (ohms)"; L "Armature Inductance (Henry)"; Kb "Back Emf constant (V.sec/rad)"; ID "Motor_ID  (#1 to #4)"
      mask help: DC motor
      mask DialogControl Container4 Prompt: Mechanical
      mask DialogControl Container9 Prompt: Electrical
      mask DialogControl Container32 Prompt: ID
      mask Display: disp('DC motor')
  DC_mot_elec1 : Subsystem  Commented=on  mask(DC motor){K=P_mot.Ka, R=P_mot.R, L=P_mot.L, Kb=P_mot.Ke, ID=P_mot.ID}
      mask prompts: K "Torque constant (N.m/A)"; R "Armature resistance (ohms)"; L "Armature Inductance (Henry)"; Kb "Back Emf constant (V.sec/rad)"; ID "Motor_ID  (#1 to #4)"
      mask help: DC motor
      mask DialogControl Container4 Prompt: Mechanical
      mask DialogControl Container9 Prompt: Electrical
      mask DialogControl Container32 Prompt: ID
      mask Display: disp('DC motor')
  Mux1 : Mux  Inputs=2
  PI_CONT : slpidlib/PID Controller  Controller=PI  Form=Parallel  TimeDomain=Continuous-time  UseExternalTs=off  SampleTime=-1  IntegratorMethod=Forward Euler  FilterMethod=Forward Euler  ControllerParametersSource=internal  P=2.97678216835849  I=24.9655384194189  D=-0.0417302954853434  UseFilter=on  N=6.67624174583517  TunerSelectOption=Transfer Function Based (PID Tuner App)  InitialConditionSource=internal  InitialConditionForIntegrator=0  InitialConditionForFilter=0  DifferentiatorICPrevScaledInput=0  ExternalReset=none  TrackingMode=off  Kt=1  LimitOutput=off  SatLimitsSource=internal  UpperSaturationLimit=inf  LowerSaturationLimit=-inf  LinearizeAsGain=on  AntiWindupMode=none  Kb=1  POutMin=[]  POutMax=[]  IOutMin=[]  IOutMax=[]  DOutMin=[]  DOutMax=[]  NOutMin=[]  NOutMax=[]  SumOutMin=[]  SumOutMax=[]  SaturationOutMin=[]  SaturationOutMax=[]  PParamMin=[]  PParamMax=[]  IParamMin=[]  IParamMax=[]  DParamMin=[]  DParamMax=[]  NParamMin=[]  NParamMax=[]  KbParamMin=[]  KbParamMax=[]  KtParamMin=[]  KtParamMax=[]  KbOutMin=[]  KbOutMax=[]  KtOutMin=[]  KtOutMax=[]  IntegratorOutMin=[]  IntegratorOutMax=[]  FilterOutMin=[]  FilterOutMax=[]  SumI1OutMin=[]  SumI1OutMax=[]  SumI2OutMin=[]  SumI2OutMax=[]  SumI3OutMin=[]  SumI3OutMax=[]  SumI4OutMin=[]  SumI4OutMax=[]  SumDOutMin=[]  SumDOutMax=[]  DifferentiatorOutMin=[]  DifferentiatorOutMax=[]  FilterDiffOutCoefMin=[]  FilterDiffOutCoefMax=[]  ReciprocalOutMin=[]  ReciprocalOutMax=[]  SumDenOutMin=[]  SumDenOutMax=[]  SumNumOutMin=[]  SumNumOutMax=[]  DivideOutMin=[]  DivideOutMax=[]  UdiffTsProdOutMin=[]  UdiffTsProdOutMax=[]  NTsProdOutMin=[]  NTsProdOutMax=[]  UintegralTsProdOutMin=[]  UintegralTsProdOutMax=[]  UngainTsProdOutMin=[]  UngainTsProdOutMax=[]  IntegratorContinuousStateAttributes=''  IntegratorStateMustResolveToSignalObject=off  IntegratorRTWStateStorageClass=Auto  FilterContinuousStateAttributes=''  FilterStateMustResolveToSignalObject=off  FilterRTWStateStorageClass=Auto  ParallelPVariant=InternalParameters  IdealPVariant=Disabled  IVariant=InternalParameters  DVariant=Disabled  IntegratorVariant=Continuous  SatVariant=Disabled  AWVariant=Passthrough  PCopyVariant=Disabled  TRVariant=Disabled  FdbkBlocksVariant=Forward  IdealPFdbkVariant=Disabled  SatFdbkVariant=Disabled  DerivativeFilterVariant=Disabled  NVariant=Disabled  NCopyVariant=Disabled_SignalSpec  FilterICVariant=Disabled  IntegratorICVariant=InternalICs  ExternalResetVariant=Disabled  TRSumVariant=Passthrough  SumFdbkVariant=Disabled  SumVariant=Sum_PI  TsampFilterVariant=InternalTs  TsampNgainVariant=Passthrough  TsampIntegralVariant=Passthrough  ExternalSaturationOutDataTypeStr=Inherit: Same as second input
  PS-Simulink Converter : nesl_utility/PS-Simulink Converter  PhysicalDomain=network_engine_domain  SubClassName=ps_output  LeftPortType=input  RightPortType=output  PseudoPeriodic=off  Frequencies=[]  Unit=rad/s  AffineConversion=off
      settings: SourceProductBaseCode=PW,SS
  PS-Simulink Converter1 : nesl_utility/PS-Simulink Converter  PhysicalDomain=network_engine_domain  SubClassName=ps_output  LeftPortType=input  RightPortType=output  PseudoPeriodic=off  Frequencies=[]  Unit=N*m  AffineConversion=off
      settings: SourceProductBaseCode=PW,SS
  Scope : Scope
  Simulink-PS Converter2 : nesl_utility/Simulink-PS Converter  PhysicalDomain=network_engine_domain  SubClassName=ps_input  LeftPortType=input  RightPortType=output  PseudoPeriodic=off  Frequencies=[]  NoiseDistribution=none  NoiseParameters=[]  Unit=V  AffineConversion=off  FilteringAndDerivatives=provide  SimscapeFilterOrder=1  InputFilterTimeConstant=0.001  UdotUserProvided=0
      settings: SourceProductBaseCode=PW,SS
  Sum1 : Sum  Inputs=|+-
  VOLTAGE Saturation : Saturate  UpperLimit=P_elec.V_mot_max  LowerLimit=P_elec.V_mot_min
      settings: AttributesFormatString=|
      | Vmax = %<UpperLimit>
      | Vmin = %<LowerLimit>
  VOLTS : Scope
  Ki : PMIOPort  Side=Right
  W_MEAS : PMIOPort  Port=2  Side=Left
  TQ_Ki : Outport  VectorParamsAs1DForOutWhenUnconnected=off
  wires:
  VOLTAGE Saturation/1 -> Simulink-PS Converter2/1, VOLTS/1  "VOLTS"
  Sum1/1 -> PI_CONT/1
  PI_CONT/1 -> VOLTAGE Saturation/1  "VOLTS"
  w_CMD_signed/1 -> Sum1/1, [w_signed]  "w_rad_per_sec"
  PS-Simulink Converter/1 -> [wM], Sum1/2
  PS-Simulink Converter1/1 -> TQ_Ki/1
  Mux1/1 -> Scope/1
  [w_signed] -> Mux1/1
  [wM] -> Mux1/2
  connections:
  Simulink-PS Converter2/RConn1 -- DC_mot_elec/LConn1
  PS-Simulink Converter1/LConn1 -- Ki/RConn1 -- DC_mot_elec/RConn1
  W_MEAS/RConn1 -- DC_mot_elec/LConn2 -- PS-Simulink Converter/LConn1

== system bh_compare_hand_to_SM_quad_pend/MODEL_SYS/bh_6DOF (Simscape)/Propellers/MOT_AERO_PROP_2/DRAQ_and_Thrust_on_PROP ==
  note: The "-1" is because DRAG is in the opposite direction
      | to the propeller SPIN direction
  PS Gain : fl_lib/Physical Signals/Functions/PS Gain  gain=-1
      settings: AttributesFormatString=GAIN= %<gain>
  PS Gain1 : fl_lib/Physical Signals/Functions/PS Gain  gain=P_one_prop.TWIST_per_w2 N*m/((rad/s)^2)
      settings: AttributesFormatString=GAIN= %<gain>
  PS Gain3 : fl_lib/Physical Signals/Functions/PS Gain  gain=P_one_prop.LIFT_per_w2 N/((rad/s)^2)
      settings: AttributesFormatString=GAIN= %<gain>
  PS Product : fl_lib/Physical Signals/Functions/PS Product
  PS Product1 : fl_lib/Physical Signals/Functions/PS Product
  PS Product2 : fl_lib/Physical Signals/Functions/PS Product
  PS Sign : fl_lib/Physical Signals/Nonlinear Operators/PS Sign
      settings: SourceProductBaseCode=SS  InternalSimscapePortConfiguration="{\"Bottom\":[],\"Left\":[{\"id\":\"I\",\"label\":\"\",\"type\":\"input\"}],\"Right\":[{\"id\":\"O\",\"label\":\"\",\"type\":\"output\"}],\"Top\":[]}"
  PS-Simulink Converter1 : nesl_utility/PS-Simulink Converter  PhysicalDomain=network_engine_domain  SubClassName=ps_output  LeftPortType=input  RightPortType=output  PseudoPeriodic=off  Frequencies=[]  Unit=N  AffineConversion=off
      settings: SourceProductBaseCode=PW,SS
  W : PMIOPort  Side=Left
  THRUST : PMIOPort  Port=2  Side=Right
  DRAQ_TQ : PMIOPort  Port=3  Side=Right
  TH_veh : Outport  VectorParamsAs1DForOutWhenUnconnected=off
  wires:
  PS-Simulink Converter1/1 -> TH_veh/1
  connections:
  PS Gain/LConn1 -- PS Sign/RConn1
  W/RConn1 -- PS Product/LConn1 -- PS Product/LConn2 -- PS Product2/LConn1 -- PS Product2/LConn2 -- PS Sign/LConn1
  PS Product/RConn1 -- PS Gain1/LConn1
  PS Gain1/RConn1 -- PS Product1/LConn2
  PS Gain/RConn1 -- PS Product1/LConn1
  DRAQ_TQ/RConn1 -- PS Product1/RConn1
  PS Product2/RConn1 -- PS Gain3/LConn1
  THRUST/RConn1 -- PS Gain3/RConn1 -- PS-Simulink Converter1/LConn1

== system bh_compare_hand_to_SM_quad_pend/MODEL_SYS/bh_6DOF (Simscape)/Propellers/MOT_AERO_PROP_2/TQ_on_propeller ==
  note: ATTENTION:
      | This subsystem computes the Torque that is applied to the
      | PROPELLER ... and NOT the torque applied to the airframe
  w_CMD_signed : Inport
  DC_mot_elec : Subsystem  mask(DC motor){K=P_mot.Ka, R=P_mot.R, L=P_mot.L, Kb=P_mot.Ke, ID=P_mot.ID}
      mask prompts: K "Torque constant (N.m/A)"; R "Armature resistance (ohms)"; L "Armature Inductance (Henry)"; Kb "Back Emf constant (V.sec/rad)"; ID "Motor_ID  (#1 to #4)"
      mask help: DC motor
      mask DialogControl Container4 Prompt: Mechanical
      mask DialogControl Container9 Prompt: Electrical
      mask DialogControl Container32 Prompt: ID
      mask Display: disp('DC motor')
  DC_mot_elec1 : Subsystem  Commented=on  mask(DC motor){K=P_mot.Ka, R=P_mot.R, L=P_mot.L, Kb=P_mot.Ke, ID=P_mot.ID}
      mask prompts: K "Torque constant (N.m/A)"; R "Armature resistance (ohms)"; L "Armature Inductance (Henry)"; Kb "Back Emf constant (V.sec/rad)"; ID "Motor_ID  (#1 to #4)"
      mask help: DC motor
      mask DialogControl Container4 Prompt: Mechanical
      mask DialogControl Container9 Prompt: Electrical
      mask DialogControl Container32 Prompt: ID
      mask Display: disp('DC motor')
  Mux1 : Mux  Inputs=2
  PI_CONT : slpidlib/PID Controller  Controller=PI  Form=Parallel  TimeDomain=Continuous-time  UseExternalTs=off  SampleTime=-1  IntegratorMethod=Forward Euler  FilterMethod=Forward Euler  ControllerParametersSource=internal  P=2.97678216835849  I=24.9655384194189  D=-0.0417302954853434  UseFilter=on  N=6.67624174583517  TunerSelectOption=Transfer Function Based (PID Tuner App)  InitialConditionSource=internal  InitialConditionForIntegrator=0  InitialConditionForFilter=0  DifferentiatorICPrevScaledInput=0  ExternalReset=none  TrackingMode=off  Kt=1  LimitOutput=off  SatLimitsSource=internal  UpperSaturationLimit=inf  LowerSaturationLimit=-inf  LinearizeAsGain=on  AntiWindupMode=none  Kb=1  POutMin=[]  POutMax=[]  IOutMin=[]  IOutMax=[]  DOutMin=[]  DOutMax=[]  NOutMin=[]  NOutMax=[]  SumOutMin=[]  SumOutMax=[]  SaturationOutMin=[]  SaturationOutMax=[]  PParamMin=[]  PParamMax=[]  IParamMin=[]  IParamMax=[]  DParamMin=[]  DParamMax=[]  NParamMin=[]  NParamMax=[]  KbParamMin=[]  KbParamMax=[]  KtParamMin=[]  KtParamMax=[]  KbOutMin=[]  KbOutMax=[]  KtOutMin=[]  KtOutMax=[]  IntegratorOutMin=[]  IntegratorOutMax=[]  FilterOutMin=[]  FilterOutMax=[]  SumI1OutMin=[]  SumI1OutMax=[]  SumI2OutMin=[]  SumI2OutMax=[]  SumI3OutMin=[]  SumI3OutMax=[]  SumI4OutMin=[]  SumI4OutMax=[]  SumDOutMin=[]  SumDOutMax=[]  DifferentiatorOutMin=[]  DifferentiatorOutMax=[]  FilterDiffOutCoefMin=[]  FilterDiffOutCoefMax=[]  ReciprocalOutMin=[]  ReciprocalOutMax=[]  SumDenOutMin=[]  SumDenOutMax=[]  SumNumOutMin=[]  SumNumOutMax=[]  DivideOutMin=[]  DivideOutMax=[]  UdiffTsProdOutMin=[]  UdiffTsProdOutMax=[]  NTsProdOutMin=[]  NTsProdOutMax=[]  UintegralTsProdOutMin=[]  UintegralTsProdOutMax=[]  UngainTsProdOutMin=[]  UngainTsProdOutMax=[]  IntegratorContinuousStateAttributes=''  IntegratorStateMustResolveToSignalObject=off  IntegratorRTWStateStorageClass=Auto  FilterContinuousStateAttributes=''  FilterStateMustResolveToSignalObject=off  FilterRTWStateStorageClass=Auto  ParallelPVariant=InternalParameters  IdealPVariant=Disabled  IVariant=InternalParameters  DVariant=Disabled  IntegratorVariant=Continuous  SatVariant=Disabled  AWVariant=Passthrough  PCopyVariant=Disabled  TRVariant=Disabled  FdbkBlocksVariant=Forward  IdealPFdbkVariant=Disabled  SatFdbkVariant=Disabled  DerivativeFilterVariant=Disabled  NVariant=Disabled  NCopyVariant=Disabled_SignalSpec  FilterICVariant=Disabled  IntegratorICVariant=InternalICs  ExternalResetVariant=Disabled  TRSumVariant=Passthrough  SumFdbkVariant=Disabled  SumVariant=Sum_PI  TsampFilterVariant=InternalTs  TsampNgainVariant=Passthrough  TsampIntegralVariant=Passthrough  ExternalSaturationOutDataTypeStr=Inherit: Same as second input
  PS-Simulink Converter : nesl_utility/PS-Simulink Converter  PhysicalDomain=network_engine_domain  SubClassName=ps_output  LeftPortType=input  RightPortType=output  PseudoPeriodic=off  Frequencies=[]  Unit=rad/s  AffineConversion=off
      settings: SourceProductBaseCode=PW,SS
  PS-Simulink Converter1 : nesl_utility/PS-Simulink Converter  PhysicalDomain=network_engine_domain  SubClassName=ps_output  LeftPortType=input  RightPortType=output  PseudoPeriodic=off  Frequencies=[]  Unit=N*m  AffineConversion=off
      settings: SourceProductBaseCode=PW,SS
  Scope : Scope
  Simulink-PS Converter2 : nesl_utility/Simulink-PS Converter  PhysicalDomain=network_engine_domain  SubClassName=ps_input  LeftPortType=input  RightPortType=output  PseudoPeriodic=off  Frequencies=[]  NoiseDistribution=none  NoiseParameters=[]  Unit=V  AffineConversion=off  FilteringAndDerivatives=provide  SimscapeFilterOrder=1  InputFilterTimeConstant=0.001  UdotUserProvided=0
      settings: SourceProductBaseCode=PW,SS
  Sum1 : Sum  Inputs=|+-
  VOLTAGE Saturation : Saturate  UpperLimit=P_elec.V_mot_min  LowerLimit=-1*P_elec.V_mot_max
      settings: AttributesFormatString=|
      | Vmax = %<UpperLimit>
      | Vmin = %<LowerLimit>
  VOLTS : Scope
  Ki : PMIOPort  Side=Right
  W_MEAS : PMIOPort  Port=2  Side=Left
  TQ_Ki : Outport  VectorParamsAs1DForOutWhenUnconnected=off
  wires:
  VOLTAGE Saturation/1 -> Simulink-PS Converter2/1, VOLTS/1  "VOLTS"
  Sum1/1 -> PI_CONT/1
  PI_CONT/1 -> VOLTAGE Saturation/1  "VOLTS"
  w_CMD_signed/1 -> Sum1/1, [w_signed]  "w_rad_per_sec"
  PS-Simulink Converter/1 -> [wM], Sum1/2
  PS-Simulink Converter1/1 -> TQ_Ki/1
  Mux1/1 -> Scope/1
  [w_signed] -> Mux1/1
  [wM] -> Mux1/2
  connections:
  DC_mot_elec/LConn1 -- Simulink-PS Converter2/RConn1
  PS-Simulink Converter1/LConn1 -- DC_mot_elec/RConn1 -- Ki/RConn1
  W_MEAS/RConn1 -- DC_mot_elec/LConn2 -- PS-Simulink Converter/LConn1

== system bh_compare_hand_to_SM_quad_pend/MODEL_SYS/bh_6DOF (Simscape)/Propellers/MOT_AERO_PROP_3/DRAQ_and_Thrust_on_PROP ==
  note: The "-1" is because DRAG is in the opposite direction
      | to the propeller SPIN direction
  PS Gain : fl_lib/Physical Signals/Functions/PS Gain  gain=-1
      settings: AttributesFormatString=GAIN= %<gain>
  PS Gain1 : fl_lib/Physical Signals/Functions/PS Gain  gain=P_one_prop.TWIST_per_w2 N*m/((rad/s)^2)
      settings: AttributesFormatString=GAIN= %<gain>
  PS Gain3 : fl_lib/Physical Signals/Functions/PS Gain  gain=P_one_prop.LIFT_per_w2 N/((rad/s)^2)
      settings: AttributesFormatString=GAIN= %<gain>
  PS Product : fl_lib/Physical Signals/Functions/PS Product
  PS Product1 : fl_lib/Physical Signals/Functions/PS Product
  PS Product2 : fl_lib/Physical Signals/Functions/PS Product
  PS Sign : fl_lib/Physical Signals/Nonlinear Operators/PS Sign
      settings: SourceProductBaseCode=SS  InternalSimscapePortConfiguration="{\"Bottom\":[],\"Left\":[{\"id\":\"I\",\"label\":\"\",\"type\":\"input\"}],\"Right\":[{\"id\":\"O\",\"label\":\"\",\"type\":\"output\"}],\"Top\":[]}"
  PS-Simulink Converter1 : nesl_utility/PS-Simulink Converter  PhysicalDomain=network_engine_domain  SubClassName=ps_output  LeftPortType=input  RightPortType=output  PseudoPeriodic=off  Frequencies=[]  Unit=N  AffineConversion=off
      settings: SourceProductBaseCode=PW,SS
  W : PMIOPort  Side=Left
  THRUST : PMIOPort  Port=2  Side=Right
  DRAQ_TQ : PMIOPort  Port=3  Side=Right
  TH_veh : Outport  VectorParamsAs1DForOutWhenUnconnected=off
  wires:
  PS-Simulink Converter1/1 -> TH_veh/1
  connections:
  PS Gain/LConn1 -- PS Sign/RConn1
  W/RConn1 -- PS Product/LConn1 -- PS Product/LConn2 -- PS Product2/LConn1 -- PS Product2/LConn2 -- PS Sign/LConn1
  PS Product/RConn1 -- PS Gain1/LConn1
  PS Gain1/RConn1 -- PS Product1/LConn2
  PS Gain/RConn1 -- PS Product1/LConn1
  DRAQ_TQ/RConn1 -- PS Product1/RConn1
  PS Product2/RConn1 -- PS Gain3/LConn1
  THRUST/RConn1 -- PS Gain3/RConn1 -- PS-Simulink Converter1/LConn1
